simulink model "DSimulator_ur10_3DOF"  (Simulink 9.0)
settings: Solver=ode1  StartTime=0.0  StopTime=30  FixedStep=0.001  RelTol=1e-3  EnableMultiTasking=on
undefined symbols (not defined in the file or in its folder): Dinamic_ur10_3DOF, SimpleRobotPlotROS
settings Model: SuppressorTable=22 serialization::archive 11 0 6 0 0 0 11 0  Creator=E. Dean  LastModifiedBy=nirnai
settings DataIOCC: LimitDataPoints=on  SignalLoggingSaveFormat=ModelDataLogs
settings OptimizationCC: ExpressionDepthLimit=2147483647
settings DebuggingCC: SolverPrmCheckMsg=warning  FcnCallInpInsideContextMsg=warning  AllowSymbolicDim=off  StateNameClashWarn=warning
settings GRTTargetCC: CombineOutputUpdateFcns=off  GRTInterface=on

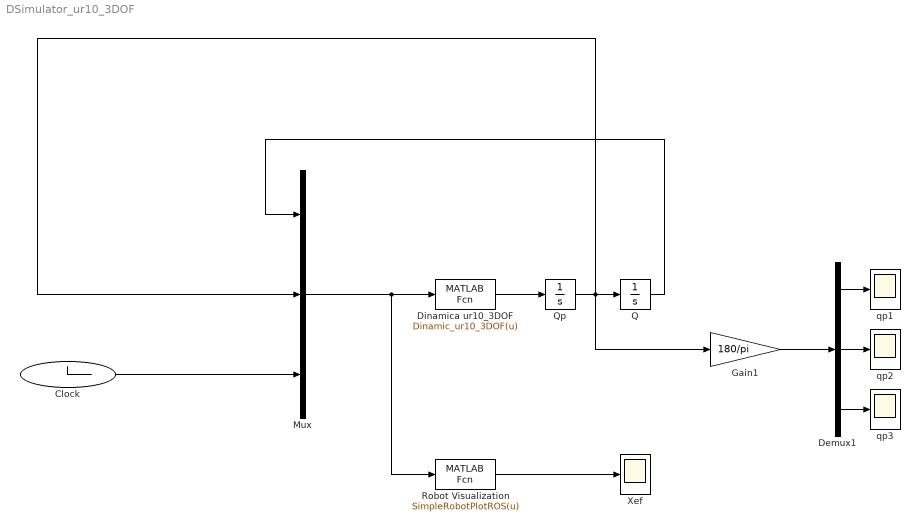
== system DSimulator_ur10_3DOF ==
  Clock : Clock
  Demux1 : Demux  Outputs=3
  Dinamica ur10_3DOF : MATLABFcn  MATLABFcn=Dinamic_ur10_3DOF(u)  OutputDimensions=3
  Gain1 : Gain  Gain=180/pi
  Mux : Mux  Inputs=3
  Q : Integrator  InitialCondition=[0;-pi/2;0]
  Qp : Integrator  InitialCondition=[0;0;0]
  Robot Visualization : MATLABFcn  MATLABFcn=SimpleRobotPlotROS(u)  OutputDimensions=3
  Xef : Scope
  qp1 : Scope
  qp2 : Scope
  qp3 : Scope
  wires:
  Qp/1 -> Mux/2, Gain1/1, Q/1
  Dinamica ur10_3DOF/1 -> Qp/1
  Q/1 -> Mux/1
  Mux/1 -> Robot Visualization/1, Dinamica ur10_3DOF/1
  Gain1/1 -> Demux1/1
  Demux1/1 -> qp1/1
  Demux1/2 -> qp2/1
  Demux1/3 -> qp3/1
  Clock/1 -> Mux/3
  Robot Visualization/1 -> Xef/1
